simulink model "sim1"  (R2019a)
settings: Solver=ode45  StartTime=0.0  StopTime=2  MaxStep=0.01  RelTol=1e-3
settings Model: Creator=Guestmit  LastModifiedBy=Guestmit

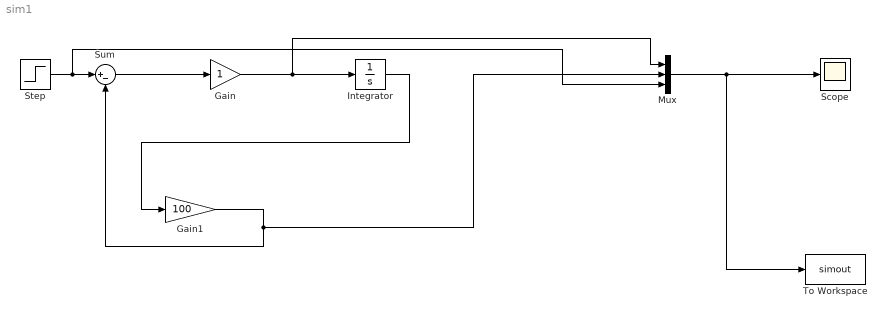
== system sim1 ==
  Gain : Gain
  Gain1 : Gain  Gain=100
  Integrator : Integrator
  Mux : Mux  Inputs=3
  Scope : Scope
  Step : Step  SampleTime=0
  Sum : Sum  Inputs=|+-
  To Workspace : ToWorkspace  VariableName=simout  SaveFormat=Timeseries  SampleTime=-1
  wires:
  Step/1 -> Mux/3, Sum/1
  Sum/1 -> Gain/1
  Integrator/1 -> Gain1/1
  Mux/1 -> Scope/1, To Workspace/1
  Gain/1 -> Mux/1, Integrator/1
  Gain1/1 -> Sum/2, Mux/2
